simulink model "ESD_Simulink11"  (R2024a)
settings: Solver=VariableStepAuto  StartTime=0.0  StopTime=70700.0  RelTol=1e-3
libraries: simulink x9
settings Model: Creator=HP  LastModifiedBy=HP

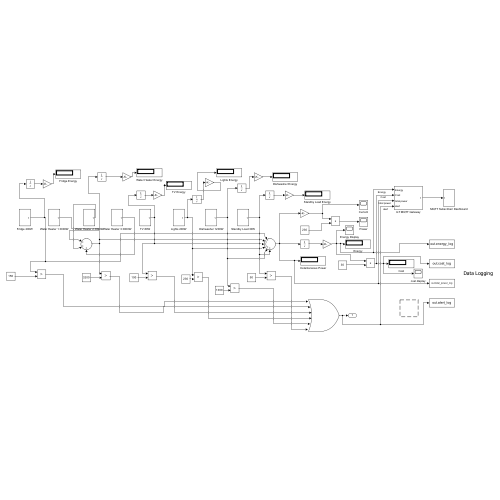
[thumbnail: Simulink's stored preview of the top-level diagram]
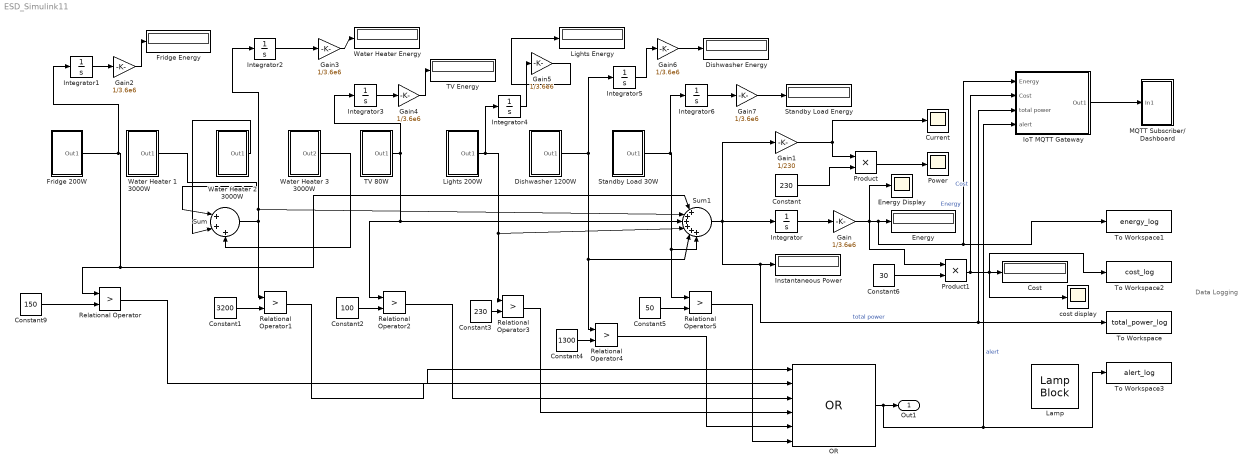
== system ESD_Simulink11 ==
  note: Data Logging
  " Dishwasher 1200W" : Subsystem
  Constant : Constant  Value=230
  Constant1 : Constant  Value=3200
  Constant2 : Constant  Value=100
  Constant3 : Constant  Value=230
  Constant4 : Constant  Value=1300
  Constant5 : Constant  Value=50
  Constant6 : Constant  Value=30
  Constant9 : Constant  Value=150
  Cost : Display
  Current : Scope
  Dishwasher Energy : Display
  Energy : Display
  Energy Display : Scope
  Fridge 200W : Subsystem
  Fridge Energy : Display
  Gain{,2..7} (7 alike) : Gain  Gain=1/3.6e6
  Gain1 : Gain  Gain=1/230
  Instantaneous Power : Display
  Integrator{,1..6} (7 alike) : Integrator
  IoT MQTT Gateway : Subsystem
  Lamp : LampBlock  LabelPosition=Bottom
  Lights 200W : Subsystem
  Lights Energy : Display
  MQTT Subscriber/ Dashboard : Subsystem
  OR : Logic  Operator=OR  Inputs=6  IconShape=distinctive  AllPortsSameDT=off  OutDataTypeStr=boolean
  Power : Scope
  Product : Product
  Product1 : Product
  Relational Operator{,1..5} (6 alike) : RelationalOperator  Operator=>  OutDataTypeStr=boolean  RndMeth=Simplest  InputSameDT=off
  Standby Load 30W : Subsystem
  Standby Load Energy : Display
  Sum : Sum  Inputs=|+++
  Sum1 : Sum  Inputs=|++++++
  TV 80W : Subsystem
  TV Energy : Display
  To Workspace : ToWorkspace  VariableName=total_power_log  SaveFormat=Timeseries  SampleTime=-1
      settings: MaxDataPoints=10000
  To Workspace1 : ToWorkspace  VariableName=energy_log  SaveFormat=Timeseries  SampleTime=-1
      settings: MaxDataPoints=10000
  To Workspace2 : ToWorkspace  VariableName=cost_log  SaveFormat=Timeseries  SampleTime=-1
      settings: MaxDataPoints=10000
  To Workspace3 : ToWorkspace  VariableName=alert_log  SaveFormat=Timeseries  SampleTime=-1
      settings: MaxDataPoints=10000
  Water Heater 1 3000W : Subsystem
  Water Heater 2 3000W : Subsystem
  Water Heater 3 3000W : Subsystem
  Water Heater Energy : Display
  cost display : Scope
  Out1 : Outport
  wires:
  Water Heater 1 3000W/1(Out1) -> Sum/1
  Water Heater 2 3000W/1(Out1) -> Sum/2
  Water Heater 3 3000W/1(Out2) -> Sum/3
  Fridge 200W/1(Out1) -> Integrator1/1, Relational Operator/1, Sum1/1
  Sum1/1 -> IoT MQTT Gateway/3(total power), To Workspace/1, Instantaneous Power/1, Integrator/1, Gain1/1  "total power"
  Integrator/1 -> Gain/1
  Gain/1 -> Product1/1, Energy Display/1, IoT MQTT Gateway/1(Energy), To Workspace1/1, Energy/1  "Energy"
  Gain1/1 -> Current/1, Product/1
  Constant/1 -> Product/2
  Product/1 -> Power/1
  Constant9/1 -> Relational Operator/2
  Constant1/1 -> Relational Operator1/2
  Constant2/1 -> Relational Operator2/2
  Constant5/1 -> Relational Operator5/2
  Constant4/1 -> Relational Operator4/2
  Constant3/1 -> Relational Operator3/2
  Relational Operator/1 -> OR/1
  Relational Operator1/1 -> OR/2
  Relational Operator2/1 -> OR/3
  Relational Operator3/1 -> OR/4
  Relational Operator4/1 -> OR/5
  Relational Operator5/1 -> OR/6
  OR/1 -> IoT MQTT Gateway/4(alert), To Workspace3/1, Out1/1  "alert"
  Integrator1/1 -> Gain2/1
  Gain2/1 -> Fridge Energy/1
  Gain3/1 -> Water Heater Energy/1
  Sum/1 -> Relational Operator1/1, Sum1/2, Integrator2/1
  Integrator2/1 -> Gain3/1
  Gain4/1 -> TV Energy/1
  TV 80W/1(Out1) -> Integrator3/1, Relational Operator2/1, Sum1/3
  Integrator3/1 -> Gain4/1
  Gain5/1 -> Lights Energy/1
  Lights 200W/1(Out1) -> Relational Operator3/1, Sum1/4, Integrator4/1
  Integrator4/1 -> Gain5/1
  Gain6/1 -> Dishwasher Energy/1
  " Dishwasher 1200W"/1(Out1) -> Integrator5/1, Relational Operator4/1, Sum1/5
  Integrator5/1 -> Gain6/1
  Gain7/1 -> Standby Load Energy/1
  Standby Load 30W/1(Out1) -> Integrator6/1, Relational Operator5/1, Sum1/6
  Integrator6/1 -> Gain7/1
  Constant6/1 -> Product1/2
  Product1/1 -> IoT MQTT Gateway/2(Cost), cost display/1, To Workspace2/1, Cost/1  "Cost"
  IoT MQTT Gateway/1(Out1) -> MQTT Subscriber/ Dashboard/1(In1)

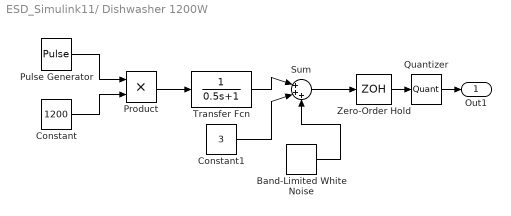
== system ESD_Simulink11/ Dishwasher 1200W ==
  Band-Limited White Noise : simulink/Sources/Band-Limited White Noise  Cov=[0.1]  Ts=0.1  seed=[23341]
  Constant : Constant  Value=1200
  Constant1 : Constant  Value=3
  Product : Product
  Pulse Generator : DiscretePulseGenerator  PulseType=Time based  Period=86400  PulseWidth=6.25  PhaseDelay=75600
  Quantizer : Quantizer  QuantizationInterval=0.2
  Sum : Sum  Inputs=|+++
  Transfer Fcn : TransferFcn  Denominator=[0.5 1]
  Zero-Order Hold : ZeroOrderHold  SampleTime=0.1
  Out1 : Outport
  wires:
  Pulse Generator/1 -> Product/1
  Constant/1 -> Product/2
  Quantizer/1 -> Out1/1
  Zero-Order Hold/1 -> Quantizer/1
  Sum/1 -> Zero-Order Hold/1
  Transfer Fcn/1 -> Sum/1
  Product/1 -> Transfer Fcn/1
  Constant1/1 -> Sum/2
  Band-Limited White Noise/1 -> Sum/3

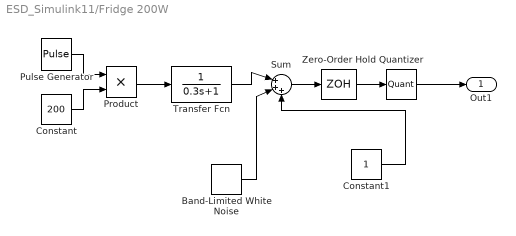
== system ESD_Simulink11/Fridge 200W ==
  Band-Limited White Noise : simulink/Sources/Band-Limited White Noise  Cov=[0.1]  Ts=0.1  seed=[23341]
  Constant : Constant  Value=200
  Constant1 : Constant
  Product : Product
  Pulse Generator : DiscretePulseGenerator  PulseType=Time based  Period=1800  PulseWidth=20
  Quantizer : Quantizer  QuantizationInterval=0.1
  Sum : Sum  Inputs=|+++
  Transfer Fcn : TransferFcn  Denominator=[0.3 1]
  Zero-Order Hold : ZeroOrderHold  SampleTime=0.1
  Out1 : Outport
  wires:
  Pulse Generator/1 -> Product/1
  Constant/1 -> Product/2
  Sum/1 -> Zero-Order Hold/1
  Zero-Order Hold/1 -> Quantizer/1
  Quantizer/1 -> Out1/1
  Product/1 -> Transfer Fcn/1
  Transfer Fcn/1 -> Sum/1
  Constant1/1 -> Sum/3
  Band-Limited White Noise/1 -> Sum/2

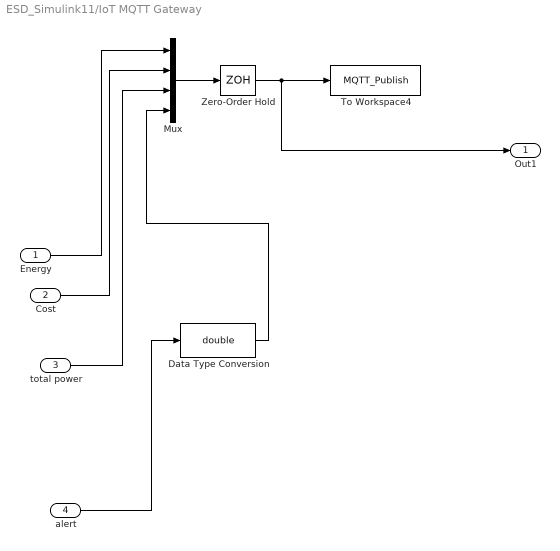
== system ESD_Simulink11/IoT MQTT Gateway ==
  Energy : Inport
  Cost : Inport  Port=2
  total power : Inport  Port=3
  alert : Inport  Port=4
  Data Type Conversion : DataTypeConversion  OutDataTypeStr=double  SaturateOnIntegerOverflow=off  RndMeth=Floor
  Mux : Mux
  To Workspace4 : ToWorkspace  VariableName=MQTT_Publish  SaveFormat=Timeseries  SampleTime=-1
  Zero-Order Hold : ZeroOrderHold  SampleTime=5
  Out1 : Outport
  wires:
  Energy/1 -> Mux/1
  Zero-Order Hold/1 -> Out1/1, To Workspace4/1
  Mux/1 -> Zero-Order Hold/1
  Cost/1 -> Mux/2
  total power/1 -> Mux/3
  alert/1 -> Data Type Conversion/1
  Data Type Conversion/1 -> Mux/4

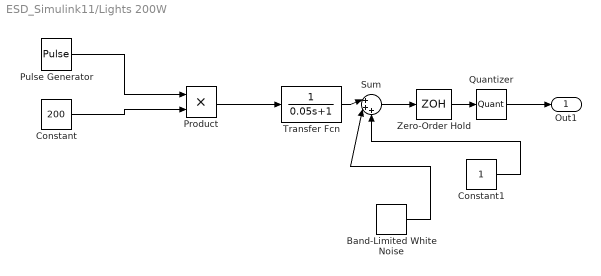
== system ESD_Simulink11/Lights 200W ==
  Band-Limited White Noise : simulink/Sources/Band-Limited White Noise  Cov=[0.1]  Ts=0.1  seed=[23341]
  Constant : Constant  Value=200
  Constant1 : Constant
  Product : Product
  Pulse Generator : DiscretePulseGenerator  PulseType=Time based  Period=86400  PulseWidth=20.8333  PhaseDelay=64800
  Quantizer : Quantizer  QuantizationInterval=0.1
  Sum : Sum  Inputs=|+++
  Transfer Fcn : TransferFcn  Denominator=[0.05 1]
  Zero-Order Hold : ZeroOrderHold
  Out1 : Outport
  wires:
  Pulse Generator/1 -> Product/1
  Constant/1 -> Product/2
  Transfer Fcn/1 -> Sum/1
  Quantizer/1 -> Out1/1
  Zero-Order Hold/1 -> Quantizer/1
  Product/1 -> Transfer Fcn/1
  Constant1/1 -> Sum/3
  Band-Limited White Noise/1 -> Sum/2
  Sum/1 -> Zero-Order Hold/1

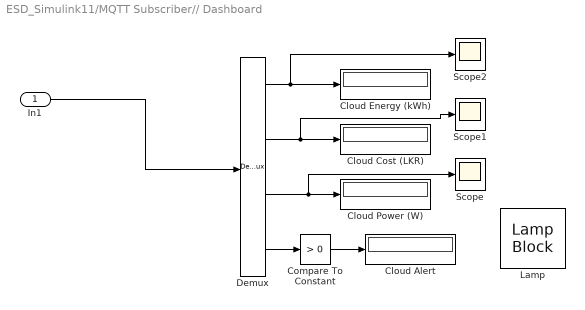
== system ESD_Simulink11/MQTT Subscriber// Dashboard ==
  In1 : Inport
  Cloud Alert : Display
  Cloud Cost (LKR) : Display
  Cloud Energy (kWh) : Display
  Cloud Power (W) : Display
  Compare To Constant : simulink/Logic and Bit Operations/Compare To Constant  relop=>  const=0  OutDataTypeStr=boolean
  Demux : Demux
  Lamp : LampBlock  LabelPosition=Hide
  Scope : Scope
  Scope1 : Scope
  Scope2 : Scope
  wires:
  Demux/2 -> Scope1/1, Cloud Cost (LKR)/1
  Demux/3 -> Scope/1, Cloud Power (W)/1
  In1/1 -> Demux/1
  Demux/4 -> Compare To Constant/1
  Demux/1 -> Scope2/1, Cloud Energy (kWh)/1
  Compare To Constant/1 -> Cloud Alert/1

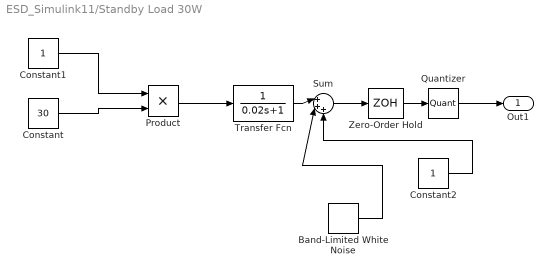
== system ESD_Simulink11/Standby Load 30W ==
  Band-Limited White Noise : simulink/Sources/Band-Limited White Noise  Cov=[0.25]  Ts=0.1  seed=[23341]
  Constant : Constant  Value=30
  Constant1 : Constant
  Constant2 : Constant
  Product : Product
  Quantizer : Quantizer  QuantizationInterval=0.05
  Sum : Sum  Inputs=|+++
  Transfer Fcn : TransferFcn  Denominator=[0.02 1]
  Zero-Order Hold : ZeroOrderHold
  Out1 : Outport
  wires:
  Constant1/1 -> Product/1
  Constant/1 -> Product/2
  Transfer Fcn/1 -> Sum/1
  Quantizer/1 -> Out1/1
  Zero-Order Hold/1 -> Quantizer/1
  Product/1 -> Transfer Fcn/1
  Constant2/1 -> Sum/3
  Band-Limited White Noise/1 -> Sum/2
  Sum/1 -> Zero-Order Hold/1

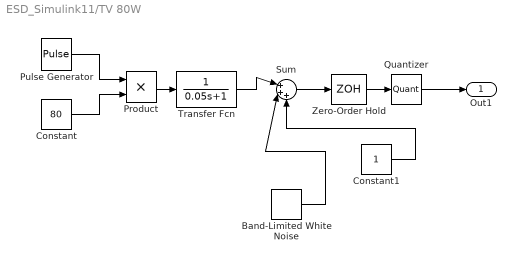
== system ESD_Simulink11/TV 80W ==
  Band-Limited White Noise : simulink/Sources/Band-Limited White Noise  Cov=[0.25]  Ts=0.1  seed=[23341]
  Constant : Constant  Value=80
  Constant1 : Constant
  Product : Product
  Pulse Generator : DiscretePulseGenerator  PulseType=Time based  Period=86400  PulseWidth=16.6667  PhaseDelay=68400
  Quantizer : Quantizer  QuantizationInterval=0.1
  Sum : Sum  Inputs=|+++
  Transfer Fcn : TransferFcn  Denominator=[0.05 1]
  Zero-Order Hold : ZeroOrderHold
  Out1 : Outport
  wires:
  Pulse Generator/1 -> Product/1
  Constant/1 -> Product/2
  Transfer Fcn/1 -> Sum/1
  Quantizer/1 -> Out1/1
  Zero-Order Hold/1 -> Quantizer/1
  Product/1 -> Transfer Fcn/1
  Constant1/1 -> Sum/3
  Band-Limited White Noise/1 -> Sum/2
  Sum/1 -> Zero-Order Hold/1

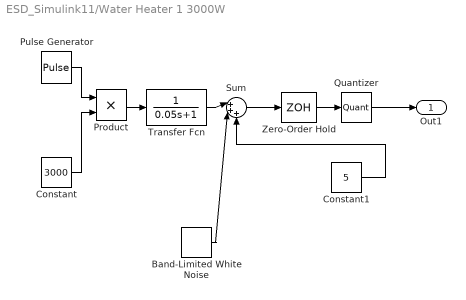
== system ESD_Simulink11/Water Heater 1 3000W ==
  Band-Limited White Noise : simulink/Sources/Band-Limited White Noise  Cov=[0.1]  Ts=0.1  seed=[23341]
  Constant : Constant  Value=3000
  Constant1 : Constant  Value=5
  Product : Product
  Pulse Generator : DiscretePulseGenerator  PulseType=Time based  Period=86400  PulseWidth=1.3889  PhaseDelay=21600
  Quantizer : Quantizer
  Sum : Sum  Inputs=|+++
  Transfer Fcn : TransferFcn  Denominator=[0.05 1]
  Zero-Order Hold : ZeroOrderHold
  Out1 : Outport
  wires:
  Pulse Generator/1 -> Product/1
  Constant/1 -> Product/2
  Sum/1 -> Zero-Order Hold/1
  Quantizer/1 -> Out1/1
  Product/1 -> Transfer Fcn/1
  Zero-Order Hold/1 -> Quantizer/1
  Transfer Fcn/1 -> Sum/1
  Constant1/1 -> Sum/3
  Band-Limited White Noise/1 -> Sum/2

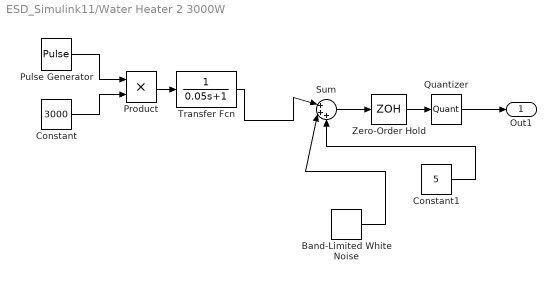
== system ESD_Simulink11/Water Heater 2 3000W ==
  Band-Limited White Noise : simulink/Sources/Band-Limited White Noise  Cov=[0.1]  Ts=0.1  seed=[23341]
  Constant : Constant  Value=3000
  Constant1 : Constant  Value=5
  Product : Product
  Pulse Generator : DiscretePulseGenerator  PulseType=Time based  Period=86400  PulseWidth=1.3889  PhaseDelay=46800
  Quantizer : Quantizer
  Sum : Sum  Inputs=|+++
  Transfer Fcn : TransferFcn  Denominator=[0.05 1]
  Zero-Order Hold : ZeroOrderHold
  Out1 : Outport
  wires:
  Pulse Generator/1 -> Product/1
  Constant/1 -> Product/2
  Transfer Fcn/1 -> Sum/1
  Quantizer/1 -> Out1/1
  Zero-Order Hold/1 -> Quantizer/1
  Product/1 -> Transfer Fcn/1
  Constant1/1 -> Sum/3
  Band-Limited White Noise/1 -> Sum/2
  Sum/1 -> Zero-Order Hold/1

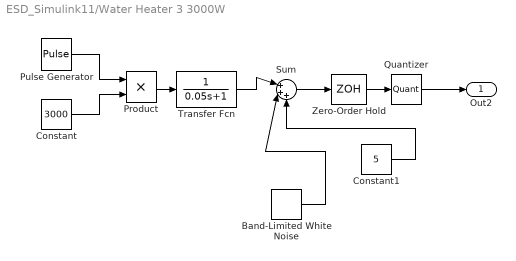
== system ESD_Simulink11/Water Heater 3 3000W ==
  Band-Limited White Noise : simulink/Sources/Band-Limited White Noise  Cov=[0.1]  Ts=0.1  seed=[23341]
  Constant : Constant  Value=3000
  Constant1 : Constant  Value=5
  Product : Product
  Pulse Generator : DiscretePulseGenerator  PulseType=Time based  Period=86400  PulseWidth=1.3889  PhaseDelay=68400
  Quantizer : Quantizer
  Sum : Sum  Inputs=|+++
  Transfer Fcn : TransferFcn  Denominator=[0.05 1]
  Zero-Order Hold : ZeroOrderHold
  Out2 : Outport
  wires:
  Pulse Generator/1 -> Product/1
  Constant/1 -> Product/2
  Transfer Fcn/1 -> Sum/1
  Quantizer/1 -> Out2/1
  Zero-Order Hold/1 -> Quantizer/1
  Product/1 -> Transfer Fcn/1
  Constant1/1 -> Sum/3
  Band-Limited White Noise/1 -> Sum/2
  Sum/1 -> Zero-Order Hold/1
